simulink model "quadplane_sim_conf"  (R2023a)
settings: Solver=FixedStepAuto  StartTime=0.0  StopTime=100  FixedStep=0.001  RelTol=1e-9
undefined symbols (not defined in the file or in its folder): Aircraft, datetime, datevec, Earth, Env, Fmu, framePeriod_s, InitCond, Telem, WGS84
libraries: simulink x9, aerolibconvert2 x5, aerolibasang x3, aerolibtransform2 x2, aerolibatmos2 x1, aerolibgravity2 x1, sharedtransform x1, uavutilslib x1, aerolibadyn x1, fuzblock x1, shared6dof x1
(part 5 of 5)

== matlab function quadplane_sim_conf/Vehicle/Forces and Moments/Propulsive/Forward Propulsion/Motor Dynamics ==
  data: total_voltage input; motor_kv input; motor_io input; motor_r input; motor_cmd input; torque_Nm output; rotational_rate input
function torque_Nm = motor(total_voltage, motor_kv, motor_io, motor_r, motor_cmd, rotational_rate)
% Calculates the torque by the motor based on rotational rate and throttle
% cmd

% Effective voltage is essentially throttle % of total voltage supplied to
% the motor. This is used as input to the motor.
% https://electronics.stackexchange.com/questions/354155/what-does-changing
% -the-throttle-to-a-bldc-esc-actually-do
effective_voltage = motor_cmd * total_voltage;
kv = motor_kv * 2 * pi / 60;

% Look at simulations/references/motor_prop.pdf
inner_term = (effective_voltage - rotational_rate / kv) / motor_r;
torque_Nm = (inner_term - motor_io) / kv;

end

== matlab function quadplane_sim_conf/Vehicle/Forces and Moments/Propulsive/Forward Propulsion/Propeller Dynamics ==
  data: airspeed input; moment_Nm output; density input; prop_rotational_rate input; thrust_N output; diameter_in input; ct_fit input; cp_fit input
function [moment_Nm, thrust_N]  = propeller(airspeed, density, prop_rotational_rate, diameter_in, ct_fit, cp_fit)
% Calculating thrust and torque from the motor

% manually converting in to m. (convlength is not supported for some reason.)
prop_radius = diameter_in * 0.0254 / 2;

% Advance ratio of propeller
lambda = airspeed / (prop_rotational_rate * prop_radius);

% thrust coefficient
ct = polyval(ct_fit, lambda);
% power coefficient
cp = polyval(cp_fit, lambda);

thrust_N = 0.5 * density * prop_rotational_rate^2 * pi * prop_radius^4 * ct;
moment_Nm = 0.5 * density * prop_rotational_rate^2 * pi * prop_radius^5 * cp;

end

== matlab function quadplane_sim_conf/Vehicle/Forces and Moments/Propulsive/Hover Propulsion/Motor Model ==
  data: motor_thrust output; poly_thrust input; poly_torque input; dir input; align input; forward_bool input; Fxyz_motor output; Motor_cmd input; Mxyz_motor output
function [motor_thrust,Fxyz_motor,Mxyz_motor] = motor_model(poly_thrust, poly_torque, dir, align, forward_bool, Motor_cmd)

% Motor commands (only for hover)
% Thrust and torque polynomial fits based on input throttle (0-1)
% 1-by-5 thrust and torques

motor_thrust  = polyval(poly_thrust,Motor_cmd);
motor_torque  = polyval(poly_torque,Motor_cmd);

% neglecting the forward motor's contribution
motor_thrust = (1 - forward_bool)' .* motor_thrust;
motor_torque = (1 - forward_bool)' .* motor_torque;

% matrix multiply with the hover motors alignment to get total thrust and
% moment
% 1-by-3 Fxyz
Fxyz_motor = motor_thrust * align;

% adding all torques based on motor spinning direction
% Dot product with negative of hover motor directions to get each motor's
% torque.
% Cross product with the motor alignment to get the torque on boxy xyz
% Returns a 1-by-3 Mxyz vector
Mxyz_motor = (motor_torque .* -dir') * abs(align);

end

== matlab function quadplane_sim_conf/Vehicle/Forces and Moments/Propulsive/Hover Propulsion/Moment From thrust arm ==
  data: cg_pos input; motor_pos input; nMotor input; align input; motor_thrust input; Mxyz_from_thrust output
function Mxyz_from_thrust = thrust_to_moment(cg_pos,motor_pos, nMotor, align, motor_thrust)
% Calculate the moment from the motors about cg.
% Returns 1-by-3 vector Mxyz

% 5-by-3 thrust from all motors in body xyz
all_motors_thrust = motor_thrust' .* align;

% calculating the moment arm for each motor
moment_arm = motor_pos - cg_pos';

moments_from_each_motor = zeros(5, 3);
Mxyz_from_thrust = zeros(1, 3);

for i = 1:nMotor

    % [Mx My Mz] for each motor
    moments_from_each_motor(i, :) = cross(moment_arm(i, :), all_motors_thrust(i, :));
    
    % [Mx My Mz] for all motors
    Mxyz_from_thrust = Mxyz_from_thrust + moments_from_each_motor(i, :);
end

end
